simulink library "RFblocks"  (R2013b)
settings: Solver=ode45  StartTime=0.0  StopTime=10.0  RelTol=1e-3
libraries: simulink_extras x1
settings Model: Creator=rmg37  LastModifiedBy=rmg37

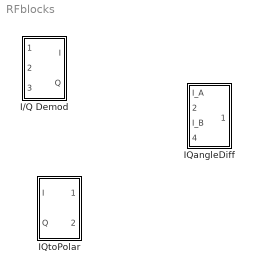
== system RFblocks ==
  I/Q Demod : Subsystem
  IQangleDiff : Subsystem
  "IQtoPolar " : Subsystem

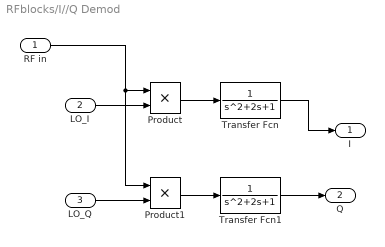
== system RFblocks/I//Q Demod ==
  RF in : Inport
  LO_I : Inport  Port=2
  "LO_Q " : Inport  Port=3
  Product : Product
  Product1 : Product
  Transfer Fcn : TransferFcn
  Transfer Fcn1 : TransferFcn
  I : Outport
  Q : Outport  Port=2
  wires:
  RF in/1 -> Product/1, Product1/1
  Transfer Fcn1/1 -> Q/1
  Product1/1 -> Transfer Fcn1/1
  "LO_Q "/1 -> Product1/2
  Transfer Fcn/1 -> I/1
  Product/1 -> Transfer Fcn/1
  LO_I/1 -> Product/2

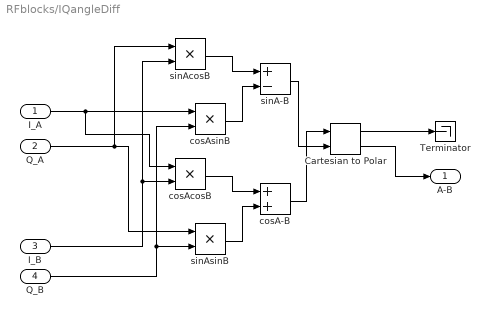
== system RFblocks/IQangleDiff ==
  I_A : Inport
  Q_A : Inport  Port=2
  I_B : Inport  Port=3
  Q_B : Inport  Port=4
  Cartesian to Polar : simulink_extras/Transformations/Cartesian to Polar
  Terminator : Terminator
  cosA-B : Sum
  cosAcosB : Product
  cosAsinB : Product
  sinA-B : Sum  Inputs=+-
  sinAcosB : Product
  sinAsinB : Product
  A-B : Outport
  wires:
  cosAcosB/1 -> cosA-B/1
  cosAsinB/1 -> sinA-B/2
  Cartesian to Polar/2 -> A-B/1
  Q_B/1 -> cosAsinB/2, sinAsinB/2
  Cartesian to Polar/1 -> Terminator/1
  I_A/1 -> cosAsinB/1, cosAcosB/1
  cosA-B/1 -> Cartesian to Polar/1
  Q_A/1 -> sinAcosB/1, sinAsinB/1
  sinAsinB/1 -> cosA-B/2
  sinA-B/1 -> Cartesian to Polar/2
  sinAcosB/1 -> sinA-B/1
  I_B/1 -> cosAcosB/2, sinAcosB/2

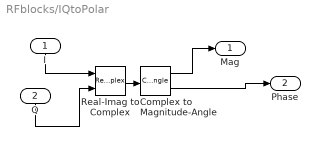
== system RFblocks/IQtoPolar  ==
  I : Inport
  Q : Inport  Port=2
  Complex to Magnitude-Angle : ComplexToMagnitudeAngle
  Real-Imag to Complex : RealImagToComplex
  Mag : Outport
  Phase : Outport  Port=2
  wires:
  Real-Imag to Complex/1 -> Complex to Magnitude-Angle/1
  Complex to Magnitude-Angle/2 -> Phase/1
  Complex to Magnitude-Angle/1 -> Mag/1
  I/1 -> Real-Imag to Complex/1
  Q/1 -> Real-Imag to Complex/2
